simulink model "husky_sim"  (R2019b)
settings: Solver=ode4  StartTime=0.0  StopTime=8  FixedStep=Ts  RelTol=1e-3
InitFcn:
  | init_model;
values from neighbouring files (symbols this model uses):
  backbone_mass_pos_wrt_body = [0.021107, -5.5457e-05, -0.041523]    [func_robot_param.m]
  del_p_FL_1 = [0.0, 0.18, 0.1]    [func_params_ext.m]
  del_p_FL_2 = [0.0, 0, 0.15]    [func_params_ext.m]
  del_y_BL = 0.125/n    (= 0.0125)    [func_params_ext.m]
  del_y_BR = 0.125/n    (= 0.0125)    [func_params_ext.m]
  del_z_BL = z_BL(2:end)-z_BL(1:n)    [func_params_ext.m]
  del_z_BR = z_BR(2:end)-z_BR(1:n)    [func_params_ext.m]
  femur_mass_loc = [2.704e-07, -0.036112, -0.082829]    [func_params_ext.m]    (also in func_robot_param.m)
  hip_orgin_wrt_backbone = [hip_FR_origin_wrt_backbone, hip_FL_origin_wrt_backbone, hip_BR_origin_wrt_backbone, hip_BL_origin_wrt_backbone].'    [func_params_ext.m]    (also in func_robot_param.m)
  leg_params = [l_hip_offset, l1, l2, l3, q_hf_offset, q_hs_offset, q_k_offset]    [func_params_ext.m]
  m = getfield(leg,'mass')    [dynamic_test.m]    (also in pen_init.m = link2.mass; test.mat = 2.2337)
  mu_s = 0.8    [func_params_ext.m]    (also in pen_init.m; test.mat)
  n = 10    [func_params_ext.m]
  p_init = p_init + 1*[0,0,0,  0,0,0,  0,-0,0,   0,0,0]    [func_params_ext.m]
  q_BL_K0 = initial_angle(12)    [func_params_ext.m]
  q_BR_K0 = initial_angle(9)    [func_params_ext.m]
  q_FL_K0 = initial_angle(6)    [func_params_ext.m]
  T_f_back_BL = 0.1/n    (= 0.01)    [func_params_ext.m]
  T_f_back_BR = 0.1/n    (= 0.01)    [func_params_ext.m]
  T_f_FL_1 = 1    [func_params_ext.m]
  T_f_FL_2 = 1    [func_params_ext.m]
  t_start = 0.32    [func_params_ext.m]
  Ts = 0.001    [func_params_ext.m]
  v_y = 0    [func_params_ext.m]
  v_z = 0    [func_params_ext.m]
undefined symbols (not defined in the file or in its folder): body, femur_left, femur_right, hip_left, hip_right, link_left, link_right, tarsus_left, tarsus_right, tibia_left, tibia_right, X, Y, Z
libraries: sm_lib x206, nesl_utility x56, dspsigops x7, Contact_Forces_Lib x4, simulink x2
(part 1 of 6)
settings Model: PauseTimes=0.4  NumberOfSteps=10  SnapshotBufferSize=100  SnapshotInterval=20  Creator=Yang  LastModifiedBy=User
settings SFSimCC: CustomCodeUndefinedFunction=UseInterfaceOnly
settings RTWCC: Description=Simulink Desktop Real-Time  SystemTargetFile=sldrt.tlc  TemplateMakefile=sldrt.tmf  RTWCompilerOptimization=on
settings CodeAppCC: MaxIdLength=95
settings SimulinkDesktopRealTimeCC: TargetPreCompLibLocation=C:\Program Files\MATLAB\R2019b\toolbox\sldrt\lib\win64  PreserveStateflowLocalDataDimensions=off
settings DiagnosticsConfigSet: SimMechanicsRigidlyBoundBlock=warning

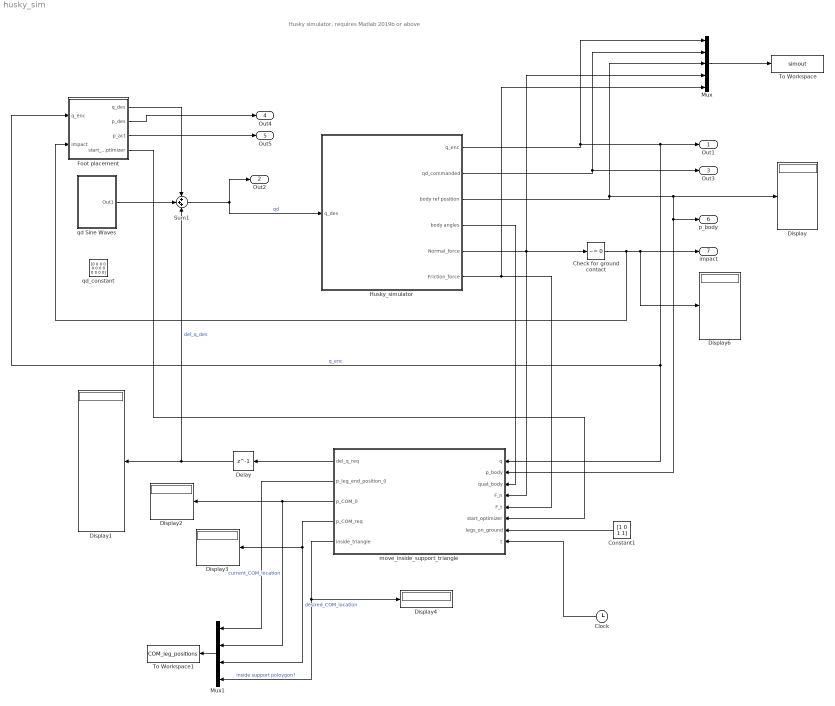
== system husky_sim ==
  note: Husky simulator, requires Matlab 2019b or above
  Check for ground contact : simulink/Logic and Bit Operations/Compare To Constant  relop=~=  const=0  OutDataTypeStr=boolean
  Clock : Clock
  Constant1 : Constant  Value=[1 0 1 1]
  Delay : Delay  DelayLength=1
  Display{,1..4,6} (6 alike) : Display
  Foot placement : Subsystem
  Husky_simulator : Subsystem
  Mux : Mux  Inputs=5
  Mux1 : Mux
  Sum1 : Sum  Inputs=3
  To Workspace : ToWorkspace  VariableName=simout  SampleTime=-1
  To Workspace1 : ToWorkspace  VariableName=COM_leg_positions  SampleTime=-1
  move_inside_support_triangle : MATLAB Function  TreatAsAtomicUnit=on
  qd Sine Waves : Subsystem
  qd_constant : Constant  Value="[0  0  0  0  0  0  0  0  0  0  0  0]"
  Out1 : Outport  SignalName=q_enc  VectorParamsAs1DForOutWhenUnconnected=off
  Out2 : Outport  Port=2  SignalName=qd  VectorParamsAs1DForOutWhenUnconnected=off
  Out3 : Outport  Port=3  SignalName=qd_commanded  VectorParamsAs1DForOutWhenUnconnected=off
  Out4 : Outport  Port=4  SignalName=p_des  VectorParamsAs1DForOutWhenUnconnected=off
  Out5 : Outport  Port=5  SignalName=p_act  VectorParamsAs1DForOutWhenUnconnected=off
  p_body : Outport  Port=6  VectorParamsAs1DForOutWhenUnconnected=off
  impact : Outport  Port=7  VectorParamsAs1DForOutWhenUnconnected=off
  wires:
  Foot placement/3(p_act) -> Out5/1
  Foot placement/2(p_des) -> Out4/1
  qd Sine Waves/1(Out1) -> Sum1/2
  Sum1/1 -> Out2/1, Husky_simulator/1(q_des)  "qd"
  Husky_simulator/2(qd_commanded) -> Out3/1, Mux/2
  Husky_simulator/5(Normal_force) -> move_inside_support_triangle/4(F_n), Mux/4, Check for ground contact/1
  Check for ground contact/1 -> Display6/1, impact/1, Foot placement/2(impact)
  Mux/1 -> To Workspace/1
  Foot placement/1(q_des) -> Sum1/1
  move_inside_support_triangle/2(p_leg_end_position_0) -> Mux1/1
  move_inside_support_triangle/5(inside_triangle) -> Mux1/4, Display4/1  "inside support poloygon?"
  move_inside_support_triangle/4(p_COM_req) -> Mux1/3, Display3/1  "desired_COM_location"
  Husky_simulator/3(body ref position) -> move_inside_support_triangle/2(p_body), p_body/1, Display/1, Mux/3
  Delay/1 -> Sum1/3, Display1/1  "del_q_des"
  move_inside_support_triangle/3(p_COM_0) -> Mux1/2, Display2/1  "current_COM_location"
  Mux1/1 -> To Workspace1/1
  move_inside_support_triangle/1(del_q_req) -> Delay/1
  Husky_simulator/4(body angles) -> move_inside_support_triangle/3(quat_body)
  Husky_simulator/1(q_enc) -> Mux/1, move_inside_support_triangle/1(q), Foot placement/1(q_enc), Out1/1  "q_enc"
  Husky_simulator/6(Friction_force) -> move_inside_support_triangle/5(F_t), Mux/5
  Foot placement/4(start_optimizer) -> move_inside_support_triangle/6(start_optimizer)
  Constant1/1 -> move_inside_support_triangle/7(legs_on_ground)
  Clock/1 -> move_inside_support_triangle/8(t)

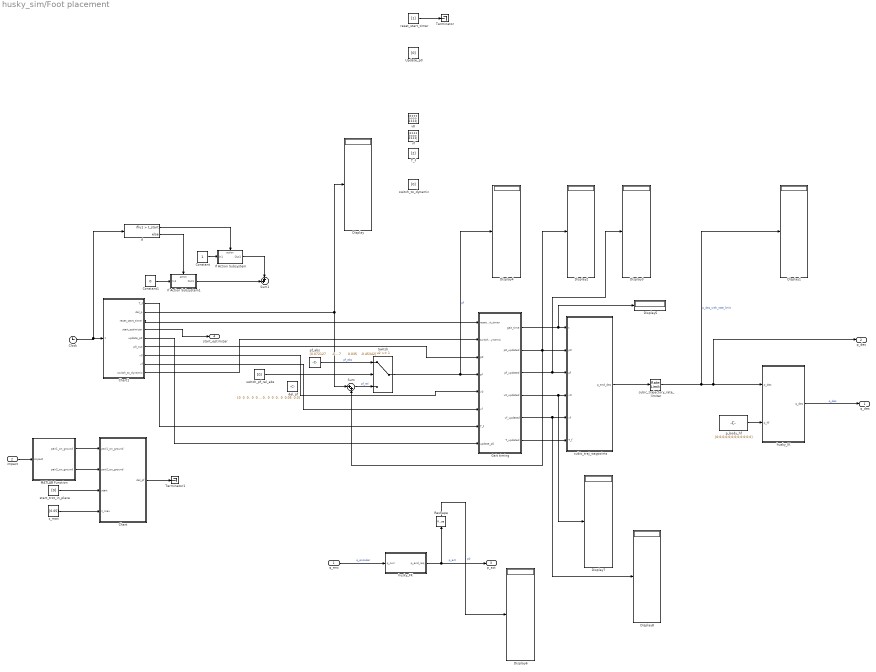
== system husky_sim/Foot placement ==
  q_enc : Inport
  impact : Inport  Port=2
  Chart : Stateflow chart  BlockKeywords=__PRM__SERIALIZED__DATA__:Stateflow Chart,Stateflow Diagram  TreatAsAtomicUnit=on
  Chart1 : Stateflow chart  BlockKeywords=__PRM__SERIALIZED__DATA__:Stateflow Chart,Stateflow Diagram  TreatAsAtomicUnit=on
  Clock : Clock
  Constant : Constant
  Constant1 : Constant  Value=0
  Display{,1..8} (9 alike) : Display
  Gait timing : Subsystem
  If : If  IfExpression=u1 > t_start
  If Action Subsystem : Subsystem  TreatAsAtomicUnit=on
  If Action Subsystem1 : Subsystem  TreatAsAtomicUnit=on
  MATLAB Function : MATLAB Function  TreatAsAtomicUnit=on
  Reshape : Reshape
  Sum : Sum  Inputs=|++
  Sum1 : Sum  Inputs=++|
  Switch : Switch  Threshold=1
  T_f : Constant  Value=[2]
  Terminator : Terminator
  Terminator1 : Terminator
  Update_p0 : Constant  Value=[0]
  cubic_traj_waypoints : MATLAB Function  TreatAsAtomicUnit=on
  cubic_trajectory_rate_limiter : RateLimiter  RisingSlewLimit=10  FallingSlewLimit=-10  SampleTimeMode=inherited
  del_pf : Constant  Value="[0  0  0,  0  0  0,  0  0  0,  0  0.05  0.0]"
  husky_FK : MATLAB Function  TreatAsAtomicUnit=on
  husky_IK : MATLAB Function  TreatAsAtomicUnit=on
  p_body_hf : Constant  Value=[0;0;0;0;0;0;0;0;0;0;0;0]
  pf_abs : Constant  Value="[0.072127      -0.035    -0.45342    0.072127       0.035    -0.45342    0.072127      -0.035    -0.45342    0.072127       0.035    -0.45342]"
  reset_start_timer : Constant  Value=[1]
  start_trot_in_place : Constant  Value=[0]
  switch_pf_rel_abs : Constant  Value=[0]
  switch_to_dynamic : Constant  Value=[0]
  v0 : Constant  Value="[0  0  0  0  0  0  0  0  0  0  0  0]"
  vf : Constant  Value="[0  0  0  0  0  0  0  0  0  0  0  0]"
  z_max : Constant  Value=[0.05]
  q_des : Outport  VectorParamsAs1DForOutWhenUnconnected=off
  p_des : Outport  Port=2  VectorParamsAs1DForOutWhenUnconnected=off
  p_act : Outport  Port=3  VectorParamsAs1DForOutWhenUnconnected=off
  start_optimizer : Outport  Port=4
  wires:
  p_body_hf/1 -> husky_IK/2(p_hf)
  cubic_traj_waypoints/1(p_end_des) -> cubic_trajectory_rate_limiter/1
  cubic_trajectory_rate_limiter/1 -> Display1/1, p_des/1, husky_IK/1(p_des)  "p_des_with_rate_limit"
  husky_IK/1(q_des) -> q_des/1  "q_des"
  q_enc/1 -> husky_FK/1(q_curr)  "q_encoder"
  husky_FK/1(p_end_req) -> p_act/1, Reshape/1  "p_act"
  Gait timing/2(p0_updated) -> Sum/2, Display2/1, cubic_traj_waypoints/2(p0)
  Gait timing/4(v0_updated) -> Display7/1, cubic_traj_waypoints/4(v0)
  Reshape/1 -> Display6/1  "p0"
  Chart1/8(vf) -> Gait timing/6(vf)
  Gait timing/5(vf_updated) -> Display8/1, cubic_traj_waypoints/5(vf)
  Chart1/7(v0) -> Gait timing/5(v0)
  switch_pf_rel_abs/1 -> Switch/2
  Switch/1 -> Display4/1, Gait timing/4(pf)  "pf"
  reset_start_timer/1 -> Terminator/1
  pf_abs/1 -> Switch/1  "pf_abs"
  Sum/1 -> Switch/3  "pf_rel"
  Gait timing/6(T_updated) -> cubic_traj_waypoints/6(T_f)
  impact/1 -> MATLAB Function/1(impact)
  MATLAB Function/1(pair1_on_ground) -> Chart/1(pair1_on_ground)
  MATLAB Function/2(pair2_on_ground) -> Chart/2(pair2_on_ground)
  start_trot_in_place/1 -> Chart/3(start)
  z_max/1 -> Chart/4(z_max)
  Chart/1(del_pf) -> Terminator1/1
  Clock/1 -> If/1, Chart1/1(t)
  Constant/1 -> If Action Subsystem/1(In1)
  If Action Subsystem/1(Out1) -> Sum1/1
  If/2 -> If Action Subsystem1/Action
  Constant1/1 -> If Action Subsystem1/1(In1)
  If Action Subsystem1/1(Out1) -> Sum1/2
  If/1 -> If Action Subsystem/Action
  Chart1/5(update_p0) -> Gait timing/8(update_p0)
  Chart1/1(T_f) -> Gait timing/7(T_f)
  Chart1/2(del_p) -> Sum/1, Display/1
  Chart1/3(reset_start_timer) -> Gait timing/1(reset_start_timer)
  Chart1/4(start_optimizer) -> start_optimizer/1
  Gait timing/3(pf_updated) -> Display3/1, cubic_traj_waypoints/3(pf)
  Gait timing/1(gait_time) -> Display5/1, cubic_traj_waypoints/1(t)
  Chart1/6(p0_out) -> Gait timing/3(p0)
  Chart1/9(switch_to_dynamic) -> Gait timing/2(switch_to_dynamic)

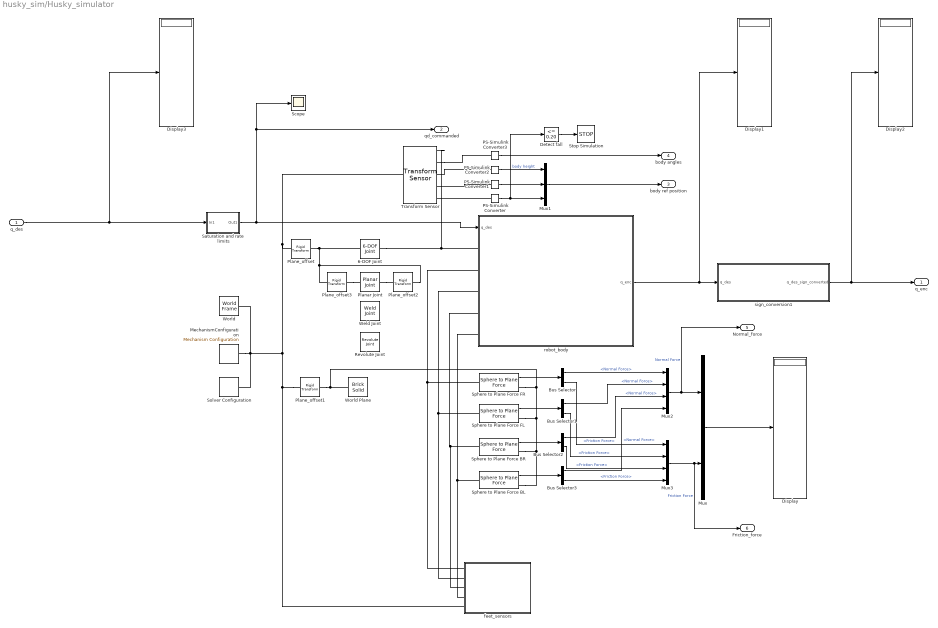
== system husky_sim/Husky_simulator ==
  q_des : Inport
  6-DOF Joint : sm_lib/Joints/6-DOF Joint  JointMode=Normal  SenseConstraintForce=off  SenseConstraintForceX=off  SenseConstraintForceY=off  SenseConstraintForceZ=off  SenseConstraintTorque=off  SenseConstraintTorqueX=off  SenseConstraintTorqueY=off  SenseConstraintTorqueZ=off  SenseTotalForce=off  SenseTotalForceX=off  SenseTotalForceY=off  SenseTotalForceZ=off  SenseTotalTorque=off  SenseTotalTorqueX=off  SenseTotalTorqueY=off  SenseTotalTorqueZ=off  CompositeWrenchDir=FollowerOnBase  CompositeWrenchFrame=BaseFrame  PxEquilibriumPosition=0  PxEquilibriumPositionUnits=m  PxSpringStiffness=0  PxSpringStiffnessUnits=N/m  PxDampingCoefficient=0  PxDampingCoefficientUnits=N/(m/s)  PxTorqueActuationMode=NoTorque  PxMotionActuationMode=ComputedMotion  PxSensePosition=off  PxSenseVelocity=off  PxSenseAcceleration=off  PxSenseTorqueForce=off  PxSenseLowerLimitTorqueForce=off  PxSenseUpperLimitTorqueForce=off  PxLowerLimitSpecify=off  PxLowerLimitBound=-1  PxLowerLimitBoundUnits=m  PxLowerLimitStiffness=1e6  PxLowerLimitStiffnessUnits=N/m  PxLowerLimitDamping=1e3  PxLowerLimitDampingUnits=N/(m/s)  PxLowerLimitTransitionRegionWidth=1e-4  PxLowerLimitTransitionRegionWidthUnits=m  PxUpperLimitSpecify=off  PxUpperLimitBound=1  PxUpperLimitBoundUnits=m  PxUpperLimitStiffness=1e6  PxUpperLimitStiffnessUnits=N/m  PxUpperLimitDamping=1e3  PxUpperLimitDampingUnits=N/(m/s)  PxUpperLimitTransitionRegionWidth=1e-4  PxUpperLimitTransitionRegionWidthUnits=m  PxPositionTargetSpecify=off  PxPositionTargetPriority=High  PxPositionTargetValue=0  PxPositionTargetValueUnits=m  PxVelocityTargetSpecify=off  PxVelocityTargetPriority=High  PxVelocityTargetValue=0  PxVelocityTargetValueUnits=m/s  PyEquilibriumPosition=0  PyEquilibriumPositionUnits=m  PySpringStiffness=0  PySpringStiffnessUnits=N/m  PyDampingCoefficient=0  PyDampingCoefficientUnits=N/(m/s)  PyTorqueActuationMode=NoTorque  PyMotionActuationMode=ComputedMotion  PySensePosition=off  PySenseVelocity=off  PySenseAcceleration=off  PySenseTorqueForce=off  PySenseLowerLimitTorqueForce=off  PySenseUpperLimitTorqueForce=off  PyLowerLimitSpecify=off  PyLowerLimitBound=-1  PyLowerLimitBoundUnits=m  PyLowerLimitStiffness=1e6  PyLowerLimitStiffnessUnits=N/m  PyLowerLimitDamping=1e3  PyLowerLimitDampingUnits=N/(m/s)  PyLowerLimitTransitionRegionWidth=1e-4  PyLowerLimitTransitionRegionWidthUnits=m  PyUpperLimitSpecify=off  PyUpperLimitBound=1  PyUpperLimitBoundUnits=m  PyUpperLimitStiffness=1e6  PyUpperLimitStiffnessUnits=N/m  PyUpperLimitDamping=1e3  PyUpperLimitDampingUnits=N/(m/s)  PyUpperLimitTransitionRegionWidth=1e-4  PyUpperLimitTransitionRegionWidthUnits=m  PyPositionTargetSpecify=off  PyPositionTargetPriority=High  PyPositionTargetValue=0  PyPositionTargetValueUnits=m  PyVelocityTargetSpecify=off  PyVelocityTargetPriority=High  PyVelocityTargetValue=0  PyVelocityTargetValueUnits=m/s  PzEquilibriumPosition=0  PzEquilibriumPositionUnits=m  PzSpringStiffness=0  PzSpringStiffnessUnits=N/m  PzDampingCoefficient=0  PzDampingCoefficientUnits=N/(m/s)  PzTorqueActuationMode=NoTorque  PzMotionActuationMode=ComputedMotion  PzSensePosition=off  PzSenseVelocity=off  PzSenseAcceleration=off  PzSenseTorqueForce=off  PzSenseLowerLimitTorqueForce=off  PzSenseUpperLimitTorqueForce=off  PzLowerLimitSpecify=off  PzLowerLimitBound=-1  PzLowerLimitBoundUnits=m  PzLowerLimitStiffness=1e6  PzLowerLimitStiffnessUnits=N/m  PzLowerLimitDamping=1e3  PzLowerLimitDampingUnits=N/(m/s)  PzLowerLimitTransitionRegionWidth=1e-4  PzLowerLimitTransitionRegionWidthUnits=m  PzUpperLimitSpecify=off  PzUpperLimitBound=1  PzUpperLimitBoundUnits=m  PzUpperLimitStiffness=1e6  PzUpperLimitStiffnessUnits=N/m  PzUpperLimitDamping=1e3  PzUpperLimitDampingUnits=N/(m/s)  PzUpperLimitTransitionRegionWidth=1e-4  PzUpperLimitTransitionRegionWidthUnits=m  PzPositionTargetSpecify=off  PzPositionTargetPriority=High  PzPositionTargetValue=0  PzPositionTargetValueUnits=m  PzVelocityTargetSpecify=off  PzVelocityTargetPriority=High  PzVelocityTargetValue=0  PzVelocityTargetValueUnits=m/s  SphDefPosRotationMethod=None  SphDefPosRotationAngleUnits=deg  SphDefPosRotationStandardAxis=+Z  SphDefPosRotationAngle=0.0  SphDefPosRotationArbitraryAxis=[0 0 1]  SphDefPosFollAlignAxisA=+X  SphDefPosBaseAlignAxisA=+Y  SphDefPosFollAlignAxisB=+Y  SphDefPosBaseAlignAxisB=+Z  SphDefPosRotationSequenceAxes=FollowerAxes  SphDefPosRotationSequence=XYX  SphDefPosRotationSequenceAngles=[0 0 0]  SphDefPosRotationSequenceAnglesUnits=deg  SphDefPosRotationMatrix=[1 0 0; 0 1 0; 0 0 1]  SphEqPosRotationMethod=None  SphEqPosRotationAngleUnits=deg  SphEqPosRotationStandardAxis=+Z  SphEqPosRotationAngle=0.0  SphEqPosRotationArbitraryAxis=[0 0 1]  SphEqPosFollAlignAxisA=+X  SphEqPosBaseAlignAxisA=+Y  SphEqPosFollAlignAxisB=+Y  SphEqPosBaseAlignAxisB=+Z  SphEqPosRotationSequenceAxes=FollowerAxes  SphEqPosRotationSequence=XYX  SphEqPosRotationSequenceAngles=[0 0 0]  SphEqPosRotationSequenceAnglesUnits=deg  SphEqPosRotationMatrix=[1 0 0; 0 1 0; 0 0 1]  SphSpringStiffness=0  SphSpringStiffnessUnits=N*m/deg  SphDampingCoefficient=0  SphDampingCoefficientUnits=N*m/(deg/s)  SphActuateTorqueX=off  SphActuateTorqueY=off  SphActuateTorqueZ=off  SphActuateTorque=off  SphTorqueActuationMode=NoTorque  SphMotionActuationMode=ComputedMotion  SphActuationFrame=BaseFrame  SphSensePosition=off  SphSenseVelocityX=off  SphSenseVelocityY=off  SphSenseVelocityZ=off  SphSenseVelocity=off  SphSenseAccelerationX=off  SphSenseAccelerationY=off  SphSenseAccelerationZ=off  SphSenseAcceleration=off  SphSenseTorqueX=off  SphSenseTorqueY=off  SphSenseTorqueZ=off  SphSenseTorqueForce=off  SphSenseLowerLimitTorqueMag=off  SphSenseUpperLimitTorqueMag=off  SphSensingFrame=BaseFrame  SphLowerLimitSpecify=off  SphLowerLimitBound=15  SphLowerLimitBoundUnits=deg  SphLowerLimitStiffness=1e4  SphLowerLimitStiffnessUnits=N*m/deg  SphLowerLimitDamping=10  SphLowerLimitDampingUnits=N*m/(deg/s)  SphLowerLimitTransitionRegionWidth=0.1  SphLowerLimitTransitionRegionWidthUnits=deg  SphUpperLimitSpecify=off  SphUpperLimitBound=45  SphUpperLimitBoundUnits=deg  SphUpperLimitStiffness=1e4  SphUpperLimitStiffnessUnits=N*m/deg  SphUpperLimitDamping=10  SphUpperLimitDampingUnits=N*m/(deg/s)  SphUpperLimitTransitionRegionWidth=0.1  SphUpperLimitTransitionRegionWidthUnits=deg  SphPositionTargetRotationMethod=None  SphPositionTargetRotationAngleUnits=deg  SphPositionTargetRotationStandardAxis=+Z  SphPositionTargetRotationAngle=0.0  SphPositionTargetRotationArbitraryAxis=[0 0 1]  SphPositionTargetFollAlignAxisA=+X  SphPositionTargetBaseAlignAxisA=+Y  SphPositionTargetFollAlignAxisB=+Y  SphPositionTargetBaseAlignAxisB=+Z  SphPositionTargetRotationSequenceAxes=FollowerAxes  SphPositionTargetRotationSequence=XYX  SphPositionTargetRotationSequenceAngles=[0 0 0]  SphPositionTargetRotationSequenceAnglesUnits=deg  SphPositionTargetRotationMatrix=[1 0 0; 0 1 0; 0 0 1]  SphPositionTargetSpecify=off  SphPositionTargetPriority=High  SphVelocityTargetValue=[0 0 0]  SphVelocityTargetValueUnits=deg/s  SphVelocityTargetSpecify=off  SphVelocityTargetPriority=High  SphVelocityTargetInFollowerFrame=on
  Bus Selector{,1..3} (4 alike) : BusSelector  OutputSignals=Normal Force,Friction Force
  Detect fall : simulink/Logic and Bit Operations/Compare To Constant  relop=<=  const=0.20  OutDataTypeStr=boolean
  Display{,1..3} (4 alike) : Display
  MechanismConfiguration : sm_lib/Utilities/Mechanism Configuration  UniformGravity=Constant  GravityVector=[0 0 -9.80665]  GravityUnits=m/s^2  LinearizationDelta=0.001
  Mux : Mux  Inputs=2
  Mux1 : Mux  Inputs=3
  Mux2 : Mux
  Mux3 : Mux
  PS-Simulink Converter{,1..3} (4 alike) : nesl_utility/PS-Simulink Converter  PhysicalDomain=network_engine_domain  SubClassName=ps_output  LeftPortType=input  RightPortType=output  PseudoPeriodic=off  Frequencies=[]  Unit=inherit  AffineConversion=off
  Planar Joint : sm_lib/Joints/Planar Joint  JointMode=Normal  SenseConstraintForce=off  SenseConstraintForceX=off  SenseConstraintForceY=off  SenseConstraintForceZ=off  SenseConstraintTorque=off  SenseConstraintTorqueX=off  SenseConstraintTorqueY=off  SenseConstraintTorqueZ=off  SenseTotalForce=off  SenseTotalForceX=off  SenseTotalForceY=off  SenseTotalForceZ=off  SenseTotalTorque=off  SenseTotalTorqueX=off  SenseTotalTorqueY=off  SenseTotalTorqueZ=off  CompositeWrenchDir=FollowerOnBase  CompositeWrenchFrame=BaseFrame  PxEquilibriumPosition=0  PxEquilibriumPositionUnits=m  PxSpringStiffness=0  PxSpringStiffnessUnits=N/m  PxDampingCoefficient=0  PxDampingCoefficientUnits=N/(m/s)  PxTorqueActuationMode=NoTorque  PxMotionActuationMode=ComputedMotion  PxSensePosition=off  PxSenseVelocity=off  PxSenseAcceleration=off  PxSenseTorqueForce=off  PxSenseLowerLimitTorqueForce=off  PxSenseUpperLimitTorqueForce=off  PxLowerLimitSpecify=off  PxLowerLimitBound=-1  PxLowerLimitBoundUnits=m  PxLowerLimitStiffness=1e6  PxLowerLimitStiffnessUnits=N/m  PxLowerLimitDamping=1e3  PxLowerLimitDampingUnits=N/(m/s)  PxLowerLimitTransitionRegionWidth=1e-4  PxLowerLimitTransitionRegionWidthUnits=m  PxUpperLimitSpecify=off  PxUpperLimitBound=1  PxUpperLimitBoundUnits=m  PxUpperLimitStiffness=1e6  PxUpperLimitStiffnessUnits=N/m  PxUpperLimitDamping=1e3  PxUpperLimitDampingUnits=N/(m/s)  PxUpperLimitTransitionRegionWidth=1e-4  PxUpperLimitTransitionRegionWidthUnits=m  PxPositionTargetSpecify=off  PxPositionTargetPriority=High  PxPositionTargetValue=0  PxPositionTargetValueUnits=m  PxVelocityTargetSpecify=off  PxVelocityTargetPriority=High  PxVelocityTargetValue=0  PxVelocityTargetValueUnits=m/s  PyEquilibriumPosition=0  PyEquilibriumPositionUnits=m  PySpringStiffness=0  PySpringStiffnessUnits=N/m  PyDampingCoefficient=0  PyDampingCoefficientUnits=N/(m/s)  PyTorqueActuationMode=NoTorque  PyMotionActuationMode=ComputedMotion  PySensePosition=off  PySenseVelocity=off  PySenseAcceleration=off  PySenseTorqueForce=off  PySenseLowerLimitTorqueForce=off  PySenseUpperLimitTorqueForce=off  PyLowerLimitSpecify=off  PyLowerLimitBound=-1  PyLowerLimitBoundUnits=m  PyLowerLimitStiffness=1e6  PyLowerLimitStiffnessUnits=N/m  PyLowerLimitDamping=1e3  PyLowerLimitDampingUnits=N/(m/s)  PyLowerLimitTransitionRegionWidth=1e-4  PyLowerLimitTransitionRegionWidthUnits=m  PyUpperLimitSpecify=off  PyUpperLimitBound=1  PyUpperLimitBoundUnits=m  PyUpperLimitStiffness=1e6  PyUpperLimitStiffnessUnits=N/m  PyUpperLimitDamping=1e3  PyUpperLimitDampingUnits=N/(m/s)  PyUpperLimitTransitionRegionWidth=1e-4  PyUpperLimitTransitionRegionWidthUnits=m  PyPositionTargetSpecify=off  PyPositionTargetPriority=High  PyPositionTargetValue=0  PyPositionTargetValueUnits=m  PyVelocityTargetSpecify=off  PyVelocityTargetPriority=High  PyVelocityTargetValue=0  PyVelocityTargetValueUnits=m/s  RzEquilibriumPosition=0  RzEquilibriumPositionUnits=deg  RzSpringStiffness=0  RzSpringStiffnessUnits=N*m/deg  RzDampingCoefficient=0  RzDampingCoefficientUnits=N*m/(deg/s)  RzTorqueActuationMode=NoTorque  RzMotionActuationMode=ComputedMotion  RzSensePosition=off  RzSenseVelocity=off  RzSenseAcceleration=off  RzSenseTorqueForce=off  RzSenseLowerLimitTorqueForce=off  RzSenseUpperLimitTorqueForce=off  RzLowerLimitSpecify=off  RzLowerLimitBound=-90  RzLowerLimitBoundUnits=deg  RzLowerLimitStiffness=1e4  RzLowerLimitStiffnessUnits=N*m/deg  RzLowerLimitDamping=10  RzLowerLimitDampingUnits=N*m/(deg/s)  RzLowerLimitTransitionRegionWidth=0.1  RzLowerLimitTransitionRegionWidthUnits=deg  RzUpperLimitSpecify=off  RzUpperLimitBound=90  RzUpperLimitBoundUnits=deg  RzUpperLimitStiffness=1e4  RzUpperLimitStiffnessUnits=N*m/deg  RzUpperLimitDamping=10  RzUpperLimitDampingUnits=N*m/(deg/s)  RzUpperLimitTransitionRegionWidth=0.1  RzUpperLimitTransitionRegionWidthUnits=deg  RzPositionTargetSpecify=off  RzPositionTargetPriority=High  RzPositionTargetValue=0  RzPositionTargetValueUnits=deg  RzVelocityTargetSpecify=off  RzVelocityTargetPriority=High  RzVelocityTargetValue=0  RzVelocityTargetValueUnits=deg/s
  Plane_offset : sm_lib/Frames and Transforms/Rigid Transform  TranslationMethod=Cartesian  TranslationStandardOffset=0  TranslationLengthUnit=m  TranslationStandardAxis=+Z  TranslationCartesianOffset=p_b0  TranslationROffset=0  TranslationROffsetUnits=m  TranslationZOffset=0  TranslationZOffsetUnits=m  TranslationThetaOffset=0  TranslationThetaOffsetUnits=deg  RotationMethod=RotationSequence  RotationAngleUnits=deg  RotationStandardAxis=+Z  RotationAngle=0.0  RotationArbitraryAxis=[0 0 1]  FollAlignAxisA=+X  BaseAlignAxisA=+Y  FollAlignAxisB=+Y  BaseAlignAxisB=+Z  RotationSequenceAxes=BaseAxes  RotationSequence=XYZ  RotationSequenceAngles=[0, 0, 0]  RotationSequenceAnglesUnits=deg  RotationMatrix=[1 0 0; 0 1 0; 0 0 1]
  Plane_offset1 : sm_lib/Frames and Transforms/Rigid Transform  TranslationMethod=Cartesian  TranslationStandardOffset=0  TranslationLengthUnit=m  TranslationStandardAxis=+Z  TranslationCartesianOffset=[0, 0, 0]  TranslationROffset=0  TranslationROffsetUnits=m  TranslationZOffset=0  TranslationZOffsetUnits=m  TranslationThetaOffset=0  TranslationThetaOffsetUnits=deg  RotationMethod=RotationSequence  RotationAngleUnits=deg  RotationStandardAxis=+Z  RotationAngle=0.0  RotationArbitraryAxis=[0 0 1]  FollAlignAxisA=+X  BaseAlignAxisA=+Y  FollAlignAxisB=+Y  BaseAlignAxisB=+Z  RotationSequenceAxes=BaseAxes  RotationSequence=XYZ  RotationSequenceAngles=[0, 0, 0]  RotationSequenceAnglesUnits=rad  RotationMatrix=[1 0 0; 0 1 0; 0 0 1]
  Plane_offset2 : sm_lib/Frames and Transforms/Rigid Transform  TranslationMethod=Cartesian  TranslationStandardOffset=0  TranslationLengthUnit=m  TranslationStandardAxis=+Z  TranslationCartesianOffset=[0, 0, 0]  TranslationROffset=0  TranslationROffsetUnits=m  TranslationZOffset=0  TranslationZOffsetUnits=m  TranslationThetaOffset=0  TranslationThetaOffsetUnits=deg  RotationMethod=RotationSequence  RotationAngleUnits=deg  RotationStandardAxis=+Z  RotationAngle=0.0  RotationArbitraryAxis=[0 0 1]  FollAlignAxisA=+X  BaseAlignAxisA=+Y  FollAlignAxisB=+Y  BaseAlignAxisB=+Z  RotationSequenceAxes=BaseAxes  RotationSequence=XYZ  RotationSequenceAngles=[-90, 0, 0]  RotationSequenceAnglesUnits=deg  RotationMatrix=[1 0 0; 0 1 0; 0 0 1]
  Plane_offset3 : sm_lib/Frames and Transforms/Rigid Transform  TranslationMethod=Cartesian  TranslationStandardOffset=0  TranslationLengthUnit=m  TranslationStandardAxis=+Z  TranslationCartesianOffset=[0, 0, 0]  TranslationROffset=0  TranslationROffsetUnits=m  TranslationZOffset=0  TranslationZOffsetUnits=m  TranslationThetaOffset=0  TranslationThetaOffsetUnits=deg  RotationMethod=RotationSequence  RotationAngleUnits=deg  RotationStandardAxis=+Z  RotationAngle=0.0  RotationArbitraryAxis=[0 0 1]  FollAlignAxisA=+X  BaseAlignAxisA=+Y  FollAlignAxisB=+Y  BaseAlignAxisB=+Z  RotationSequenceAxes=BaseAxes  RotationSequence=XYZ  RotationSequenceAngles=[90, 0, 0]  RotationSequenceAnglesUnits=deg  RotationMatrix=[1 0 0; 0 1 0; 0 0 1]
  Revolute Joint : sm_lib/Joints/Revolute Joint  JointMode=Normal  SenseConstraintForce=off  SenseConstraintForceX=off  SenseConstraintForceY=off  SenseConstraintForceZ=off  SenseConstraintTorque=off  SenseConstraintTorqueX=off  SenseConstraintTorqueY=off  SenseConstraintTorqueZ=off  SenseTotalForce=off  SenseTotalForceX=off  SenseTotalForceY=off  SenseTotalForceZ=off  SenseTotalTorque=off  SenseTotalTorqueX=off  SenseTotalTorqueY=off  SenseTotalTorqueZ=off  CompositeWrenchDir=FollowerOnBase  CompositeWrenchFrame=BaseFrame  EquilibriumPosition=0  EquilibriumPositionUnits=deg  SpringStiffness=0  SpringStiffnessUnits=N*m/deg  DampingCoefficient=0  DampingCoefficientUnits=N*m/(deg/s)  TorqueActuationMode=NoTorque  MotionActuationMode=ComputedMotion  SensePosition=off  SenseVelocity=off  SenseAcceleration=off  SenseTorqueForce=off  SenseLowerLimitTorqueForce=off  SenseUpperLimitTorqueForce=off  LowerLimitSpecify=off  LowerLimitBound=-90  LowerLimitBoundUnits=deg  LowerLimitStiffness=1e4  LowerLimitStiffnessUnits=N*m/deg  LowerLimitDamping=10  LowerLimitDampingUnits=N*m/(deg/s)  LowerLimitTransitionRegionWidth=0.1  LowerLimitTransitionRegionWidthUnits=deg  UpperLimitSpecify=off  UpperLimitBound=90  UpperLimitBoundUnits=deg  UpperLimitStiffness=1e4  UpperLimitStiffnessUnits=N*m/deg  UpperLimitDamping=10  UpperLimitDampingUnits=N*m/(deg/s)  UpperLimitTransitionRegionWidth=0.1  UpperLimitTransitionRegionWidthUnits=deg  PositionTargetSpecify=off  PositionTargetPriority=High  PositionTargetValue=0  PositionTargetValueUnits=deg  VelocityTargetSpecify=off  VelocityTargetPriority=High  VelocityTargetValue=0  VelocityTargetValueUnits=deg/s
  Saturation and rate limits : Subsystem
  Scope : Scope
  Solver Configuration : nesl_utility/Solver Configuration  PhysicalDomain=network_engine_domain  SubClassName=solver  LeftPortType=input  RightPortType=generic  Tones=[]  Harmonics=[]  SimulateNoise=off  Profile=off  UseLocalSampling=off  EnableSwitchedLinearOptims=on  FrequencyDomain=off  UseCCode=off  RelTol=0.001  AbsTol=1e-06  MinStep=1e-09  ToWorkspace=off  RevertToSquareIcSolve=off  NumHomotopyIterations=100  PhasorMode=off  PhasorModeNumHarmonics=1  DoDC=off  ResidualTolerance=1e-09  UseLocalSolver=off  LocalSolverChoice=NE_BACKWARD_EULER_ADVANCER  LocalSolverSampleTime=0.001  DoFixedCost=off  MaxNonlinIter=3  MaxModeIter=2  LinearAlgebra=auto  EquationFormulation=NE_TIME_EF  DelaysMemoryBudget=1024  AutomaticFiltering=on  FilteringTimeConstant=0.001  PartitionStorageMethod=AS_NEEDED  PartitionMemoryBudget=1024  PartitionMethod=ROBUST
  "Sphere to Plane Force BL " : Contact_Forces_Lib/3D/Sphere to Plane Force  sphere_rad=0.021  plane_lenx=5  plane_leny=5  plane_depth=0.001  force_law=Linear  k_contact=c_k  b_contact=c_b  pen_full_damp_F=1e-4  pen_exponent=1  custom_param_1=1  custom_param_2=1  friction_law=Stick-Slip Continuous  mu_kinetic=mu_k  mu_static=mu_s  v_thr=v_th  vis_on=on  vis_opc_en=0  vis_len_plaBz=0.001  vis_clr=[0.9 0.2 0.2]  vis_opc=0.7
  "Sphere to Plane Force BR " : Contact_Forces_Lib/3D/Sphere to Plane Force  sphere_rad=0.021  plane_lenx=5  plane_leny=5  plane_depth=0.001  force_law=Linear  k_contact=c_k  b_contact=c_b  pen_full_damp_F=1e-4  pen_exponent=1  custom_param_1=1  custom_param_2=1  friction_law=Stick-Slip Continuous  mu_kinetic=mu_k  mu_static=mu_s  v_thr=v_th  vis_on=off  vis_opc_en=0  vis_len_plaBz=0.001  vis_clr=[0.9 0.2 0.2]  vis_opc=0.7
  Sphere to Plane Force FL : Contact_Forces_Lib/3D/Sphere to Plane Force  sphere_rad=0.021  plane_lenx=5  plane_leny=5  plane_depth=0.001  force_law=Linear  k_contact=c_k  b_contact=c_b  pen_full_damp_F=1e-4  pen_exponent=1  custom_param_1=1  custom_param_2=1  friction_law=Stick-Slip Continuous  mu_kinetic=mu_k  mu_static=mu_s  v_thr=v_th  vis_on=off  vis_opc_en=0  vis_len_plaBz=0.001  vis_clr=[0.9 0.2 0.2]  vis_opc=0.7
  Sphere to Plane Force FR : Contact_Forces_Lib/3D/Sphere to Plane Force  sphere_rad=0.021  plane_lenx=5  plane_leny=5  plane_depth=0.001  force_law=Linear  k_contact=c_k  b_contact=c_b  pen_full_damp_F=1e-4  pen_exponent=1  custom_param_1=1  custom_param_2=1  friction_law=Stick-Slip Continuous  mu_kinetic=mu_k  mu_static=mu_s  v_thr=v_th  vis_on=off  vis_opc_en=0  vis_len_plaBz=0.001  vis_clr=[0.9 0.2 0.2]  vis_opc=0.7
  Stop Simulation : Stop
  Transform Sensor : sm_lib/Frames and Transforms/Transform Sensor  MeasurementFrame=World  SenseAngle=off  SenseAxis=off  SenseAngle1=off  SenseAngle2=off  SenseAngle3=off  SenseQ=on  SenseR=off  SenseOmegaX=off  SenseOmegaY=off  SenseOmegaZ=off  SenseOmega1=off  SenseOmega2=off  SenseOmega3=off  SenseQDot=off  SenseRDot=off  SenseAlphaX=off  SenseAlphaY=off  SenseAlphaZ=off  SenseAlpha1=off  SenseAlpha2=off  SenseAlpha3=off  SenseQDDot=off  SenseRDDot=off  SenseX=on  SenseY=on  SenseZ=on  SenseRad=off  SenseAzim=off  SenseDist=off  SenseInc=off  SenseXDot=off  SenseYDot=off  SenseZDot=off  SenseRadDot=off  SenseAzimDot=off  SenseDistDot=off  SenseIncDot=off  SenseXDDot=off  SenseYDDot=off  SenseZDDot=off  SenseRadDDot=off  SenseAzimDDot=off  SenseDistDDot=off  SenseIncDDot=off
  Weld Joint : sm_lib/Joints/Weld Joint  JointMode=Normal  SenseConstraintForce=off  SenseConstraintForceX=off  SenseConstraintForceY=off  SenseConstraintForceZ=off  SenseConstraintTorque=off  SenseConstraintTorqueX=off  SenseConstraintTorqueY=off  SenseConstraintTorqueZ=off  SenseTotalForce=off  SenseTotalForceX=off  SenseTotalForceY=off  SenseTotalForceZ=off  SenseTotalTorque=off  SenseTotalTorqueX=off  SenseTotalTorqueY=off  SenseTotalTorqueZ=off  CompositeWrenchDir=FollowerOnBase  CompositeWrenchFrame=BaseFrame
  World : sm_lib/Frames and Transforms/World Frame
  "World Plane " : sm_lib/Body Elements/Brick Solid  GraphicAmbientColor=[0.15 0.15 0.15 1.0]  BasedOnType=Density  BrickDimensions=[5 5 0.001]  BrickDimensionUnits=m  CenterOfMass=[0 0 0]  CenterOfMassUnits=m  GraphicDiffuseColor=[0.5 0.5 0.5]  Density=1000  DensityUnits=kg/m^3  DoExposeReferenceFrame=on  GraphicEmissiveColor=[0.0 0.0 0.0 1.0]  ExportEntireGeometry=off  SerializedFrames=<Frames/>  MarkerShape=Sphere  MarkerSize=10  GraphicType=FromGeometry  InertiaType=CalculateFromGeometry  Mass=1  MassUnits=kg  MomentsOfInertia=[1 1 1]  MomentsOfInertiaUnits=kg*m^2  GraphicOpacity=1.0  ProductsOfInertia=[0 0 0]  ProductsOfInertiaUnits=kg*m^2  GraphicShininess=75  GraphicSpecularColor=[0.5 0.5 0.5 1.0]  GraphicVisPropType=SimpleVisualProperties
  feet_sensors : Subsystem
  robot_body : Subsystem
  sign_conversion1 : MATLAB Function  TreatAsAtomicUnit=on
  q_enc : Outport  VectorParamsAs1DForOutWhenUnconnected=off
  qd_commanded : Outport  Port=2  VectorParamsAs1DForOutWhenUnconnected=off
  body ref position : Outport  Port=3
  body angles : Outport  Port=4
  Normal_force : Outport  Port=5
  Friction_force : Outport  Port=6
  wires:
  Saturation and rate limits/1(Out1) -> qd_commanded/1, Scope/1, robot_body/1(q_des)
  Sphere to Plane Force FR/1 -> Bus Selector/1
  Sphere to Plane Force FL/1 -> Bus Selector1/1
  "Sphere to Plane Force BR "/1 -> Bus Selector2/1
  "Sphere to Plane Force BL "/1 -> Bus Selector3/1
  Mux/1 -> Display/1
  PS-Simulink Converter/1 -> Mux1/3, Detect fall/1  "body height"
  PS-Simulink Converter2/1 -> Mux1/1
  PS-Simulink Converter1/1 -> Mux1/2
  Detect fall/1 -> Stop Simulation/1
  Mux1/1 -> body ref position/1
  Mux2/1 -> Normal_force/1, Mux/1  "Normal Force"
  Mux3/1 -> Friction_force/1, Mux/2  "Friction Force"
  Bus Selector/1 -> Mux2/1  "<Normal Force>"
  Bus Selector1/1 -> Mux2/2  "<Normal Force>"
  Bus Selector2/1 -> Mux2/3  "<Normal Force>"
  Bus Selector3/1 -> Mux2/4  "<Normal Force>"
  Bus Selector/2 -> Mux3/1  "<Friction Force>"
  Bus Selector1/2 -> Mux3/2  "<Friction Force>"
  Bus Selector2/2 -> Mux3/3  "<Friction Force>"
  Bus Selector3/2 -> Mux3/4  "<Friction Force>"
  q_des/1 -> Display3/1, Saturation and rate limits/1(In1)
  PS-Simulink Converter3/1 -> body angles/1
  robot_body/1(q_enc) -> Display1/1, sign_conversion1/1(q_des)
  sign_conversion1/1(q_des_sign_converted) -> Display2/1, q_enc/1
  connections:
  Plane_offset1/LConn1 -- feet_sensors/LConn5 -- Solver Configuration/RConn1 -- World/RConn1 -- MechanismConfiguration/RConn1 -- Transform Sensor/LConn1 -- Plane_offset/LConn1
  "Sphere to Plane Force BR "/LConn1 -- feet_sensors/LConn3 -- robot_body/LConn4
  "Sphere to Plane Force BL "/LConn1 -- feet_sensors/LConn4 -- robot_body/LConn5
  Sphere to Plane Force FR/LConn1 -- feet_sensors/LConn1 -- robot_body/LConn2
  Sphere to Plane Force FL/LConn1 -- feet_sensors/LConn2 -- robot_body/LConn3
  PS-Simulink Converter/LConn1 -- Transform Sensor/RConn5
  PS-Simulink Converter1/LConn1 -- Transform Sensor/RConn4
  PS-Simulink Converter2/LConn1 -- Transform Sensor/RConn3
  Transform Sensor/RConn1 -- robot_body/LConn1 -- 6-DOF Joint/RConn1
  Plane_offset3/RConn1 -- Planar Joint/LConn1
  Planar Joint/RConn1 -- Plane_offset2/LConn1
  Transform Sensor/RConn2 -- PS-Simulink Converter3/LConn1
  Plane_offset1/RConn1 -- "Sphere to Plane Force BL "/RConn1 -- "Sphere to Plane Force BR "/RConn1 -- Sphere to Plane Force FL/RConn1 -- Sphere to Plane Force FR/RConn1 -- "World Plane "/RConn1
  Plane_offset/RConn1 -- 6-DOF Joint/LConn1 -- Plane_offset2/RConn1 -- Plane_offset3/LConn1

== system husky_sim/qd Sine Waves ==
  Mux1 : Mux  Inputs=12
  qd Sine BL HF : Sin  Amplitude=0  Frequency=6.2832  SampleTime=0
  qd Sine BL HS : Sin  Amplitude=0  Frequency=6.2832  SampleTime=0
  qd Sine BL K : Sin  Amplitude=0  Frequency=6.2832  SampleTime=0
  qd Sine BR HF : Sin  Amplitude=0  Frequency=6.2832  SampleTime=0
  qd Sine BR HS : Sin  Amplitude=0  Frequency=6.2832  SampleTime=0
  qd Sine BR K : Sin  Amplitude=0  Frequency=6.2832  SampleTime=0
  qd Sine FL HF : Sin  Amplitude=0  Frequency=6.2832  SampleTime=0
  qd Sine FL HS : Sin  Amplitude=0  Frequency=6.2832  SampleTime=0
  qd Sine FL K : Sin  Amplitude=0  Frequency=6.2832  SampleTime=0
  qd Sine FR HF : Sin  Amplitude=0  Frequency=6.2832  SampleTime=0
  qd Sine FR HS : Sin  Amplitude=0  Frequency=6.2832  SampleTime=0
  qd Sine FR K : Sin  Amplitude=0  Frequency=6.2832  SampleTime=0
  Out1 : Outport  VectorParamsAs1DForOutWhenUnconnected=off
  wires:
  Mux1/1 -> Out1/1
  qd Sine BL K/1 -> Mux1/12
  qd Sine BR K/1 -> Mux1/9
  qd Sine BR HF/1 -> Mux1/7
  qd Sine BL HS/1 -> Mux1/11
  qd Sine BR HS/1 -> Mux1/8
  qd Sine FR HF/1 -> Mux1/1
  qd Sine FL HF/1 -> Mux1/4
  qd Sine FR HS/1 -> Mux1/2
  qd Sine FL K/1 -> Mux1/6
  qd Sine FL HS/1 -> Mux1/5
  qd Sine FR K/1 -> Mux1/3
  qd Sine BL HF/1 -> Mux1/10

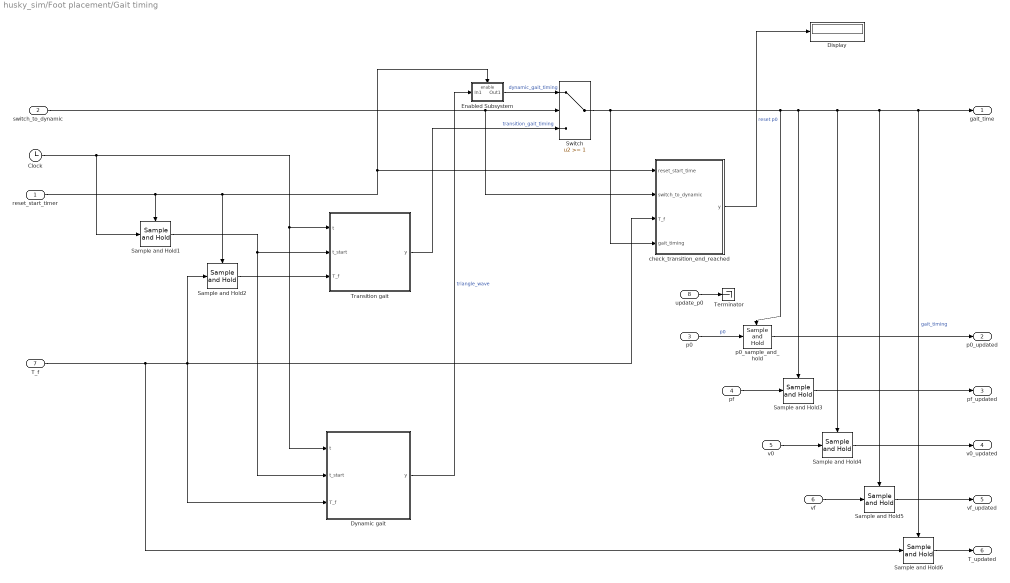
== system husky_sim/Foot placement/Gait timing ==
  reset_start_timer : Inport
  switch_to_dynamic : Inport  Port=2
  p0 : Inport  Port=3
  pf : Inport  Port=4
  v0 : Inport  Port=5
  vf : Inport  Port=6
  T_f : Inport  Port=7
  update_p0 : Inport  Port=8
  Clock : Clock
  Display : Display
  Dynamic gait : MATLAB Function  TreatAsAtomicUnit=on
  Enabled Subsystem : Subsystem  TreatAsAtomicUnit=on
  Sample and Hold1 : dspsigops/Sample and Hold  trig=Rising edge  initCond=0  latchinput=on
  Sample and Hold2 : dspsigops/Sample and Hold  trig=Rising edge  initCond=0  latchinput=on
  Sample and Hold3 : dspsigops/Sample and Hold  trig=Rising edge  initCond=[0.072127,-0.0350,-0.45342, 0.072127,0.0350,-0.45342, 0.072127,-0.0350,-0.45342 0.072127,0.0350,-0.45342]  latchinput=on
  Sample and Hold4 : dspsigops/Sample and Hold  trig=Rising edge  initCond=[0.0,0.0,0,0,0,0,0,0,0,0,0,0]  latchinput=on
  Sample and Hold5 : dspsigops/Sample and Hold  trig=Rising edge  initCond=[0.0,0.0,0,0,0,0,0,0,0,0,0,0]  latchinput=on
  Sample and Hold6 : dspsigops/Sample and Hold  trig=Rising edge  initCond=1  latchinput=on
  Switch : Switch  Threshold=1
  Terminator : Terminator
  Transition gait : MATLAB Function  TreatAsAtomicUnit=on
  check_transition_end_reached : MATLAB Function  TreatAsAtomicUnit=on
  p0_sample_and_hold : dspsigops/Sample and Hold  trig=Rising edge  initCond=p_init  latchinput=on
  gait_time : Outport  VectorParamsAs1DForOutWhenUnconnected=off
  p0_updated : Outport  Port=2  VectorParamsAs1DForOutWhenUnconnected=off
  pf_updated : Outport  Port=3  VectorParamsAs1DForOutWhenUnconnected=off
  v0_updated : Outport  Port=4  VectorParamsAs1DForOutWhenUnconnected=off
  vf_updated : Outport  Port=5  VectorParamsAs1DForOutWhenUnconnected=off
  T_updated : Outport  Port=6  VectorParamsAs1DForOutWhenUnconnected=off
  wires:
  Switch/1 -> p0_sample_and_hold/Trigger, Sample and Hold6/Trigger, gait_time/1, Sample and Hold5/Trigger, Sample and Hold4/Trigger, Sample and Hold3/Trigger, check_transition_end_reached/4(gait_timing)  "gait_timing"
  Dynamic gait/1(y) -> Enabled Subsystem/1(In1)  "triangle_wave"
  Transition gait/1(y) -> Switch/3  "transition_gait_timing"
  Sample and Hold1/1 -> Transition gait/2(t_start), Dynamic gait/2(t_start)
  Clock/1 -> Sample and Hold1/1, Transition gait/1(t), Dynamic gait/1(t)
  Sample and Hold2/1 -> Transition gait/3(T_f)
  reset_start_timer/1 -> Sample and Hold1/Trigger, Sample and Hold2/Trigger, check_transition_end_reached/1(reset_start_time), Enabled Subsystem/Enable
  switch_to_dynamic/1 -> check_transition_end_reached/2(switch_to_dynamic), Switch/2
  Enabled Subsystem/1(Out1) -> Switch/1  "dynamic_gait_timing"
  pf/1 -> Sample and Hold3/1
  Sample and Hold6/1 -> T_updated/1
  Sample and Hold3/1 -> pf_updated/1
  T_f/1 -> check_transition_end_reached/3(T_f), Sample and Hold2/1, Dynamic gait/3(T_f), Sample and Hold6/1
  Sample and Hold5/1 -> vf_updated/1
  Sample and Hold4/1 -> v0_updated/1
  p0_sample_and_hold/1 -> p0_updated/1
  v0/1 -> Sample and Hold4/1
  vf/1 -> Sample and Hold5/1
  p0/1 -> p0_sample_and_hold/1  "p0"
  check_transition_end_reached/1(y) -> Display/1  "reset p0"
  update_p0/1 -> Terminator/1

== system husky_sim/Foot placement/If Action Subsystem ==
  In1 : Inport
  Action Port : ActionPort  ActionPortLabel=if(u1 > t_start)
  Out1 : Outport
  wires:
  In1/1 -> Out1/1

== system husky_sim/Foot placement/If Action Subsystem1 ==
  In1 : Inport
  Action Port : ActionPort  ActionPortLabel=else
  Out1 : Outport
  wires:
  In1/1 -> Out1/1

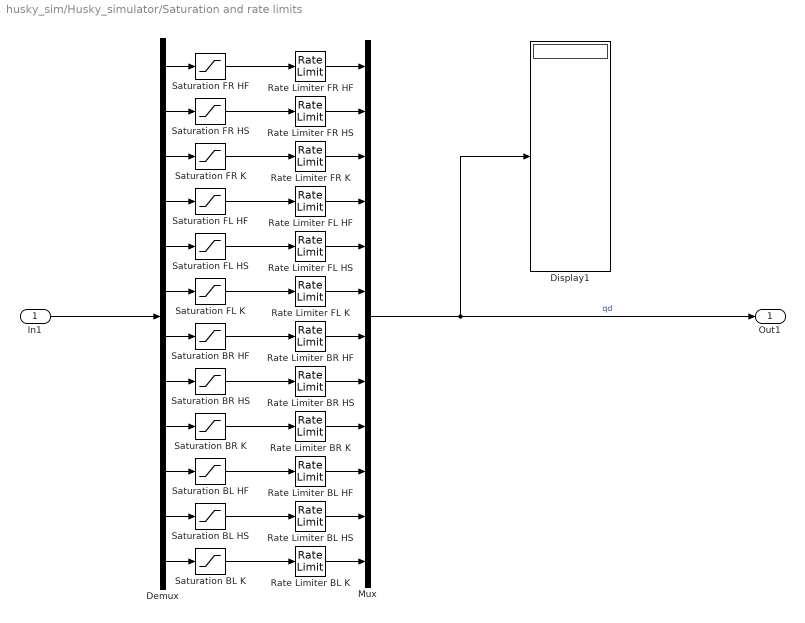
== system husky_sim/Husky_simulator/Saturation and rate limits ==
  In1 : Inport
  Demux : Demux  Outputs=12
  Display1 : Display
  Mux : Mux  Inputs=12
  Rate Limiter BL HF : RateLimiter  RisingSlewLimit=34.9066  FallingSlewLimit=-34.9066  SampleTimeMode=inherited
  Rate Limiter BL HS : RateLimiter  RisingSlewLimit=34.9066  FallingSlewLimit=-34.9066  SampleTimeMode=inherited
  Rate Limiter BL K : RateLimiter  RisingSlewLimit=34.9066  FallingSlewLimit=-34.9066  SampleTimeMode=inherited
  Rate Limiter BR HF : RateLimiter  RisingSlewLimit=34.9066  FallingSlewLimit=-34.9066  SampleTimeMode=inherited
  Rate Limiter BR HS : RateLimiter  RisingSlewLimit=34.9066  FallingSlewLimit=-34.9066  SampleTimeMode=inherited
  Rate Limiter BR K : RateLimiter  RisingSlewLimit=34.9066  FallingSlewLimit=-34.9066  SampleTimeMode=inherited
  Rate Limiter FL HF : RateLimiter  RisingSlewLimit=34.9066  FallingSlewLimit=-34.9066  SampleTimeMode=inherited
  Rate Limiter FL HS : RateLimiter  RisingSlewLimit=34.9066  FallingSlewLimit=-34.9066  SampleTimeMode=inherited
  Rate Limiter FL K : RateLimiter  RisingSlewLimit=34.9066  FallingSlewLimit=-34.9066  SampleTimeMode=inherited
  Rate Limiter FR HF : RateLimiter  RisingSlewLimit=34.9066  FallingSlewLimit=-34.9066  SampleTimeMode=inherited
  Rate Limiter FR HS : RateLimiter  RisingSlewLimit=34.9066  FallingSlewLimit=-34.9066  SampleTimeMode=inherited
  Rate Limiter FR K : RateLimiter  RisingSlewLimit=34.9066  FallingSlewLimit=-34.9066  SampleTimeMode=inherited
  Saturation BL HF : Saturate  UpperLimit=1.5708  LowerLimit=-0.5236
  Saturation BL HS : Saturate  UpperLimit=1.5708  LowerLimit=-1.5708
  Saturation BL K : Saturate  UpperLimit=1.0472  LowerLimit=-0.5236
  Saturation BR HF : Saturate  UpperLimit=1.5708  LowerLimit=-0.5236
  Saturation BR HS : Saturate  UpperLimit=1.5708  LowerLimit=-1.5708
  Saturation BR K : Saturate  UpperLimit=1.0472  LowerLimit=-0.5236
  Saturation FL HF : Saturate  UpperLimit=1.5708  LowerLimit=-0.5236
  Saturation FL HS : Saturate  UpperLimit=1.5708  LowerLimit=-1.5708
  Saturation FL K : Saturate  UpperLimit=1.0472  LowerLimit=-0.5236
  Saturation FR HF : Saturate  UpperLimit=1.5708  LowerLimit=-0.5236
  Saturation FR HS : Saturate  UpperLimit=1.5708  LowerLimit=-1.5708
  Saturation FR K : Saturate  UpperLimit=1.0472  LowerLimit=-0.5236
  Out1 : Outport  VectorParamsAs1DForOutWhenUnconnected=off
  wires:
  In1/1 -> Demux/1
  Demux/1 -> Saturation FR HF/1
  Rate Limiter FR HF/1 -> Mux/1
  Saturation FR HF/1 -> Rate Limiter FR HF/1
  Rate Limiter FR HS/1 -> Mux/2
  Demux/2 -> Saturation FR HS/1
  Rate Limiter FR K/1 -> Mux/3
  Saturation FR HS/1 -> Rate Limiter FR HS/1
  Demux/3 -> Saturation FR K/1
  Demux/4 -> Saturation FL HF/1
  Rate Limiter FL HS/1 -> Mux/5
  Demux/6 -> Saturation FL K/1
  Saturation FR K/1 -> Rate Limiter FR K/1
  Saturation FL HF/1 -> Rate Limiter FL HF/1
  Demux/5 -> Saturation FL HS/1
  Rate Limiter FL HF/1 -> Mux/4
  Saturation FL HS/1 -> Rate Limiter FL HS/1
  Rate Limiter FL K/1 -> Mux/6
  Demux/7 -> Saturation BR HF/1
  Rate Limiter BL HS/1 -> Mux/11
  Rate Limiter BL K/1 -> Mux/12
  Rate Limiter BR K/1 -> Mux/9
  Saturation BR HF/1 -> Rate Limiter BR HF/1
  Saturation BR HS/1 -> Rate Limiter BR HS/1
  Saturation BL HS/1 -> Rate Limiter BL HS/1
  Demux/8 -> Saturation BR HS/1
  Demux/12 -> Saturation BL K/1
  Saturation FL K/1 -> Rate Limiter FL K/1
  Demux/9 -> Saturation BR K/1
  Saturation BR K/1 -> Rate Limiter BR K/1
  Rate Limiter BR HS/1 -> Mux/8
  Demux/10 -> Saturation BL HF/1
  Rate Limiter BL HF/1 -> Mux/10
  Saturation BL HF/1 -> Rate Limiter BL HF/1
  Demux/11 -> Saturation BL HS/1
  Rate Limiter BR HF/1 -> Mux/7
  Saturation BL K/1 -> Rate Limiter BL K/1
  Mux/1 -> Out1/1, Display1/1  "qd"

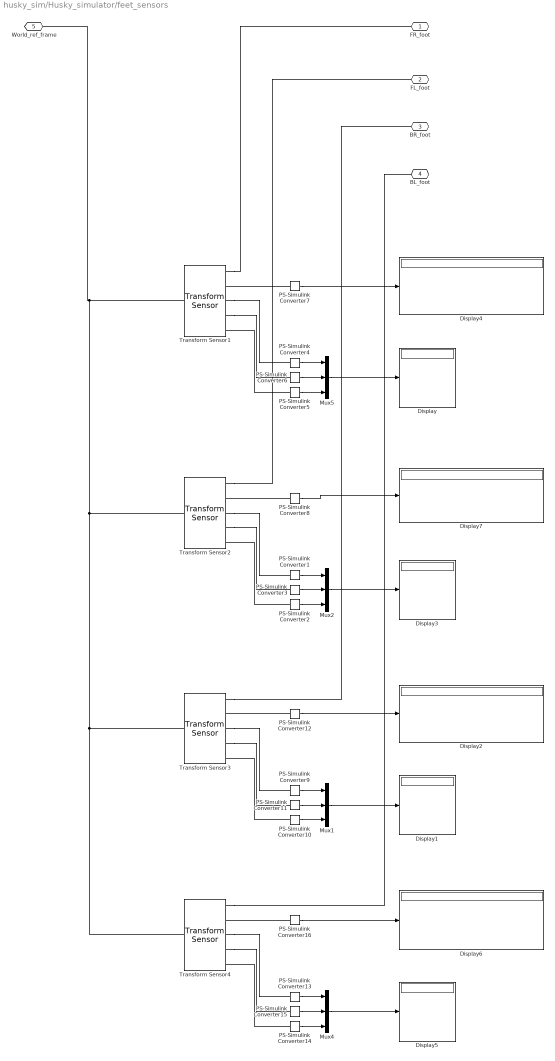
== system husky_sim/Husky_simulator/feet_sensors ==
  Display{,1..7} (8 alike) : Display
  Mux{1..2,4..5} (4 alike) : Mux  Inputs=3
  PS-Simulink Converter{1..16} (16 alike) : nesl_utility/PS-Simulink Converter  PhysicalDomain=network_engine_domain  SubClassName=ps_output  LeftPortType=input  RightPortType=output  PseudoPeriodic=off  Frequencies=[]  Unit=inherit  AffineConversion=off
  Transform Sensor{1..4} (4 alike) : sm_lib/Frames and Transforms/Transform Sensor  MeasurementFrame=World  SenseAngle=off  SenseAxis=off  SenseAngle1=off  SenseAngle2=off  SenseAngle3=off  SenseQ=off  SenseR=on  SenseOmegaX=off  SenseOmegaY=off  SenseOmegaZ=off  SenseOmega1=off  SenseOmega2=off  SenseOmega3=off  SenseQDot=off  SenseRDot=off  SenseAlphaX=off  SenseAlphaY=off  SenseAlphaZ=off  SenseAlpha1=off  SenseAlpha2=off  SenseAlpha3=off  SenseQDDot=off  SenseRDDot=off  SenseX=on  SenseY=on  SenseZ=on  SenseRad=off  SenseAzim=off  SenseDist=off  SenseInc=off  SenseXDot=off  SenseYDot=off  SenseZDot=off  SenseRadDot=off  SenseAzimDot=off  SenseDistDot=off  SenseIncDot=off  SenseXDDot=off  SenseYDDot=off  SenseZDDot=off  SenseRadDDot=off  SenseAzimDDot=off  SenseDistDDot=off  SenseIncDDot=off
  FR_foot : PMIOPort  Side=Left
  FL_foot : PMIOPort  Port=2  Side=Left
  BR_foot : PMIOPort  Port=3  Side=Left
  BL_foot : PMIOPort  Port=4  Side=Left
  World_ref_frame : PMIOPort  Port=5  Side=Left
  wires:
  Mux5/1 -> Display/1
  PS-Simulink Converter4/1 -> Mux5/1
  PS-Simulink Converter6/1 -> Mux5/2
  PS-Simulink Converter7/1 -> Display4/1
  PS-Simulink Converter5/1 -> Mux5/3
  PS-Simulink Converter14/1 -> Mux4/3
  Mux4/1 -> Display5/1
  PS-Simulink Converter15/1 -> Mux4/2
  PS-Simulink Converter16/1 -> Display6/1
  PS-Simulink Converter13/1 -> Mux4/1
  PS-Simulink Converter10/1 -> Mux1/3
  PS-Simulink Converter9/1 -> Mux1/1
  PS-Simulink Converter12/1 -> Display2/1
  PS-Simulink Converter11/1 -> Mux1/2
  Mux1/1 -> Display1/1
  PS-Simulink Converter2/1 -> Mux2/3
  PS-Simulink Converter1/1 -> Mux2/1
  PS-Simulink Converter8/1 -> Display7/1
  PS-Simulink Converter3/1 -> Mux2/2
  Mux2/1 -> Display3/1
  connections:
  Transform Sensor3/LConn1 -- Transform Sensor4/LConn1 -- Transform Sensor2/LConn1 -- Transform Sensor1/LConn1 -- World_ref_frame/RConn1
  Transform Sensor1/RConn1 -- FR_foot/RConn1
  Transform Sensor3/RConn1 -- BR_foot/RConn1
  Transform Sensor4/RConn1 -- BL_foot/RConn1
  Transform Sensor2/RConn1 -- FL_foot/RConn1
  Transform Sensor4/RConn4 -- PS-Simulink Converter15/LConn1
  PS-Simulink Converter12/LConn1 -- Transform Sensor3/RConn2
  Transform Sensor3/RConn3 -- PS-Simulink Converter9/LConn1
  Transform Sensor4/RConn3 -- PS-Simulink Converter13/LConn1
  Transform Sensor3/RConn4 -- PS-Simulink Converter11/LConn1
  PS-Simulink Converter7/LConn1 -- Transform Sensor1/RConn2
  Transform Sensor2/RConn4 -- PS-Simulink Converter3/LConn1
  Transform Sensor1/RConn4 -- PS-Simulink Converter6/LConn1
  PS-Simulink Converter10/LConn1 -- Transform Sensor3/RConn5
  PS-Simulink Converter5/LConn1 -- Transform Sensor1/RConn5
  Transform Sensor2/RConn3 -- PS-Simulink Converter1/LConn1
  PS-Simulink Converter8/LConn1 -- Transform Sensor2/RConn2
  PS-Simulink Converter16/LConn1 -- Transform Sensor4/RConn2
  PS-Simulink Converter14/LConn1 -- Transform Sensor4/RConn5
  PS-Simulink Converter2/LConn1 -- Transform Sensor2/RConn5
  Transform Sensor1/RConn3 -- PS-Simulink Converter4/LConn1

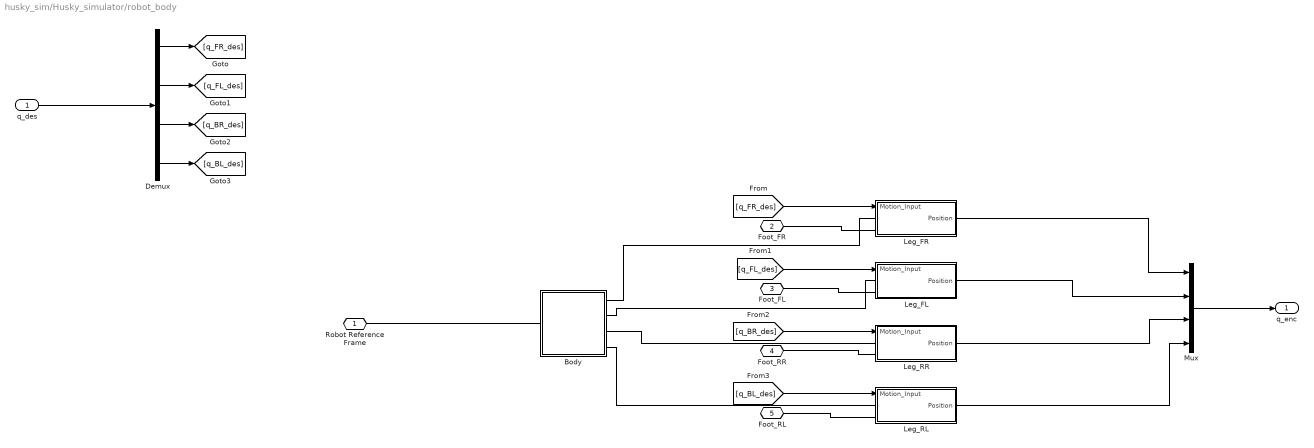
== system husky_sim/Husky_simulator/robot_body ==
  q_des : Inport
  Body : Subsystem
  Demux : Demux
  Leg_FL : Subsystem
  Leg_FR : Subsystem
  Leg_RL : Subsystem
  Leg_RR : Subsystem
  Mux : Mux
  Robot Reference Frame : PMIOPort  Side=Left
  Foot_FR : PMIOPort  Port=2  Side=Left
  Foot_FL : PMIOPort  Port=3  Side=Left
  Foot_RR : PMIOPort  Port=4  Side=Left
  Foot_RL : PMIOPort  Port=5  Side=Left
  q_enc : Outport  VectorParamsAs1DForOutWhenUnconnected=off
  wires:
  q_des/1 -> Demux/1
  Demux/1 -> [q_FR_des]
  Demux/2 -> [q_FL_des]
  Demux/3 -> [q_BR_des]
  Demux/4 -> [q_BL_des]
  Mux/1 -> q_enc/1
  Leg_RL/1(Position) -> Mux/4
  Leg_FL/1(Position) -> Mux/2
  Leg_FR/1(Position) -> Mux/1
  [q_FR_des] -> Leg_FR/1(Motion_Input)
  [q_BR_des] -> Leg_RR/1(Motion_Input)
  [q_FL_des] -> Leg_FL/1(Motion_Input)
  Leg_RR/1(Position) -> Mux/3
  [q_BL_des] -> Leg_RL/1(Motion_Input)
  connections:
  Foot_FL/RConn1 -- Leg_FL/LConn2
  Leg_RR/LConn2 -- Foot_RR/RConn1
  Body/LConn1 -- Robot Reference Frame/RConn1
  Body/RConn4 -- Leg_RL/LConn1
  Body/RConn2 -- Leg_FL/LConn1
  Body/RConn1 -- Leg_FR/LConn1
  Foot_FR/RConn1 -- Leg_FR/LConn2
  Body/RConn3 -- Leg_RR/LConn1
  Foot_RL/RConn1 -- Leg_RL/LConn2

== system husky_sim/Foot placement/Gait timing/Enabled Subsystem ==
  In1 : Inport
  Enable : EnablePort
  Out1 : Outport  VectorParamsAs1DForOutWhenUnconnected=off
  wires:
  In1/1 -> Out1/1
